simulink model "KitGewerk2_v1_4"  (R2014a)
settings: Solver=ode3  StartTime=0.0  StopTime=inf  FixedStep=0.005  RelTol=1e-3
undefined symbols (not defined in the file or in its folder): Com1, none
libraries: slrtlib x14, dspswit3 x1, xpcseriallib x1
(part 2 of 2)

== matlab function KitGewerk2_v1_4/Robotino/assemble robotino response ==
  data: v_x_in input; robotino_response output; v_y_in input; v_theta_in input; distance_measuring_sensors_in input; bumper_in input; light_barrier_in input; slider_in input
%%%%%%%%%%%%%%%%%%%%%%%%%%%%%%%%%%%%%%%%%%%%%%%%%%%%%%%%%%%%%%%%%%%%%%%%%%%
% Assembly of robot data in a vector of 34 elements.                      %
%                                                                         %
% inputs:   longitudinal, lateral and rotational velocity (in mm/s),      %
%           shaft positions of the three motors (4 elements per motor),   %
%           running times of the three motors (3 elements per motor),     %
%           values of the nine IR-sensors (in mm),                        %
%           bumper collision (1 = no collision;                           %
%                             0 = collision)                              %
% outputs:  vector containing assembled input data                        %
%%%%%%%%%%%%%%%%%%%%%%%%%%%%%%%%%%%%%%%%%%%%%%%%%%%%%%%%%%%%%%%%%%%%%%%%%%%
function robotino_response = fcn(v_x_in, v_y_in, v_theta_in, ...
                                 distance_measuring_sensors_in, ...
                                 bumper_in, light_barrier_in, slider_in)
                                 % motor_positions_in, time_bytes_in, ...)
robotino_response = [light_barrier_in, slider_in, v_x_in, v_y_in, ...
                     v_theta_in, ...%motor_positions_in, time_bytes_in, ...
                     distance_measuring_sensors_in, bumper_in]';

== matlab function KitGewerk2_v1_4/Robotino/light barrier & slider ==
  data: di03_bump_in input; light_barrier output; slider output
function [light_barrier, slider] = fcn(di03_bump_in)
%%%%%%%%%%%%%%%%%%%%%%%%%%%%%%%%%%%%%%%%%%%%%%%%%%%%%%%%%%%%%%%%%%%%%%%%%%%
% di03_bump_in = 0 alternatively 12 ->  no light barrier activation       %
%                                       no slider activation              %
% di03_bump_in = 13                 ->  only light barrier activation     %
% di03_bump_in = 14                 ->  only slider activation            %
% di03_bump_in = 15                 ->  light barrier activation          %
%                                       slider activation                 %
%%%%%%%%%%%%%%%%%%%%%%%%%%%%%%%%%%%%%%%%%%%%%%%%%%%%%%%%%%%%%%%%%%%%%%%%%%%
% function [light_barrier, slider] = fcn(di03_bump_in)
% bin = dec2bin(di03_bump_in);
% if bin(3) == 1
%     light_barrier = 1;
% else
%     light_barrier = 0;
% end
% if bin(4) == 1
%     slider = 1;
% else
%     slider = 0;
% end
if     di03_bump_in == 13
    light_barrier = 1;
    slider        = 0;
elseif di03_bump_in == 14
    light_barrier = 0;
    slider        = 1;
elseif di03_bump_in == 15
    light_barrier = 1;
    slider        = 1;
else
    light_barrier = 0;
    slider        = 0;
end

== matlab function KitGewerk2_v1_4/Begrenzung1 ==
  data: win input; wout output
function wout = fnc(win)
wert= zeros(1);
if win > 500
    wert = 500;
else
    wert = win;
end
wout = wert;

== matlab function KitGewerk2_v1_4/Begrenzung2 ==
  data: win input; wout output
function wout = fnc(win)
wert= zeros(1);
if win > 3,14
    wert = 3,14;
else
    wert = win;
end
wout = wert;

== matlab function KitGewerk2_v1_4/Gewerk_2/Kollisionserkennung ==
  data: d_Abstand input; b_stop output boolean; ad_Abstandssensor input
function b_stop = fcn(d_Abstand,ad_Abstandssensor)
b_stop=false;
if sum(isnan(ad_Abstandssensor))==9 % nan = kein Hinderniss
    % kein Hinderniss   
    b_stop= false; 
else
    % Hinderniss entdeckt, min. ein Sensor(kein nan)
    if ( (ad_Abstandssensor(1)<d_Abstand) || (ad_Abstandssensor(2)<d_Abstand) || (ad_Abstandssensor(3)<d_Abstand) || ...
         (ad_Abstandssensor(4)<d_Abstand) ||(ad_Abstandssensor(5)<d_Abstand) ||(ad_Abstandssensor(6)<d_Abstand) || ...
         (ad_Abstandssensor(7)<d_Abstand) || (ad_Abstandssensor(8)<d_Abstand) ||(ad_Abstandssensor(9)<d_Abstand)) 

    b_stop= true;
    end
end

== matlab function KitGewerk2_v1_4/Gewerk_2/Wegpunkte an Regelung bereitstellen ==
  data: ad_PL input; d_Y_soll output double; d_X_soll output double; d_Phi_soll output double; d_V_Max_soll output double; int_I input
function [d_Y_soll,d_X_soll,d_Phi_soll,d_V_Max_soll]= fcn(ad_PL,int_I)

int_I=int_I+1; %Offset, da Zeilenindex bei 1 beginnt

d_Y_soll= ad_PL(int_I,1);
d_X_soll= ad_PL(int_I,2);
d_Phi_soll= ad_PL(int_I,3);
d_V_Max_soll= ad_PL(int_I,4);

== stateflow chart KitGewerk2_v1_4/Gewerk_2/Zustandsautomat Bahnplanung ==
  state Auftrag_Warteposition/init
  note: Hier Ausgang zur Regelung
  state DStern
  state AuftragsV_AustrittKritBereich
    note: 1. Rob steht auf Schlüsselplatz
        |  -> Habe ich noch einen Auftrag?
        | ja: Weitermachen
        | nein: Melden zu GW1 und warten dann weitermachen
        | 2. Überprüfen ob Roboter im Austrittsbereich
        | 3. Bei Verlassen wird Schlüsselplatz freigegeben
  state Fahrt_in_Nav1
    state Prioritaeten erkennen und auswerten
      höchste prio
      RobMussNeuBerechnen =1 (zustand verlassen , d*)
      niedrige prio
      Warten und nach zeitspanne deadlock melden
    state Kollisionserkennung
      Bremsbit setzen
    state Mensch
      warten
      irgendwann GW1 benachrichtigen
    (default) -> Kollisionserkennung
    Kollisionserkennung -> Prioritaeten erkennen und auswerten [order 2] : robi
    Mensch -> Kollisionserkennung : weg frei
    Prioritaeten erkennen und auswerten -> Kollisionserkennung : weg wieder frei
    Kollisionserkennung -> Mensch [order 1] : kein robi
  state Schluesselplatz_Routinen
    state Nav2
      ist noch ein Fahrauftrag im auftrag enthalten?
      Wenn ja dann prüfe ob nav2 Frei
      Fahre entweder zu schlüsselplatz nav1 oder 2
    state Stationen
    state Entscheider
      Geneiere stationsnummer
      aus auftrag
    state Warteplaetze
    note: platznr>16 &&platnr<=20
    note: stationsnr>20
    state Ladestationen
    Stationen -> Nav2
    Entscheider -> Stationen [order 1] : platznr <=16
    (default) -> Entscheider
    Entscheider -> Warteplaetze [order 2]
    Entscheider -> Ladestationen [order 3]
  state Fahrt_in_Nav2
    state ?
    note: 1. Ausgänge zur Regelung
        | 2. Wegpunktlisten statisch
        | 3. Bei Eintritt Nav2 Marke entziehen
        | 4. Bei Austritt Nav2 Marke freigeben
  Auftrag_Warteposition/init -> DStern
  (default) -> Auftrag_Warteposition/init
  AuftragsV_AustrittKritBereich -> DStern [order 1] : [#Auftrag>0 && !Nav2]
  Fahrt_in_Nav1 -> DStern [order 2] : [RobMussNeuBerechnen]
  DStern -> Fahrt_in_Nav1 : [WegBerechnet]
  Schluesselplatz_Routinen -> AuftragsV_AustrittKritBereich : [Routine abgearbeitet]
  AuftragsV_AustrittKritBereich -> Fahrt_in_Nav2 [order 2] : [#Auftrag>1 && Nav2]
  Fahrt_in_Nav1 -> Schluesselplatz_Routinen [order 1] : [Schlüsselplatz erreicht]
  Fahrt_in_Nav2 -> Schluesselplatz_Routinen : [Schlüsselplatz erreicht]
  data: aintGW1send input uint32; aintGW2receive output double; ad_WPL output double; ad_Kameradaten input double; ad_Abstandssensoren input double; bStop output boolean
